simulink model "C_Sim"  (R2020b)
settings: Solver=ode4  StartTime=0.0  StopTime=t_f  FixedStep=dt  RelTol=1e-3
undefined symbols (not defined in the file or in its folder): A, B, K, Q, R, X0
settings Model: Creator=vahed  LastModifiedBy=vahed
settings DataIOCC: ReturnWorkspaceOutputs=off

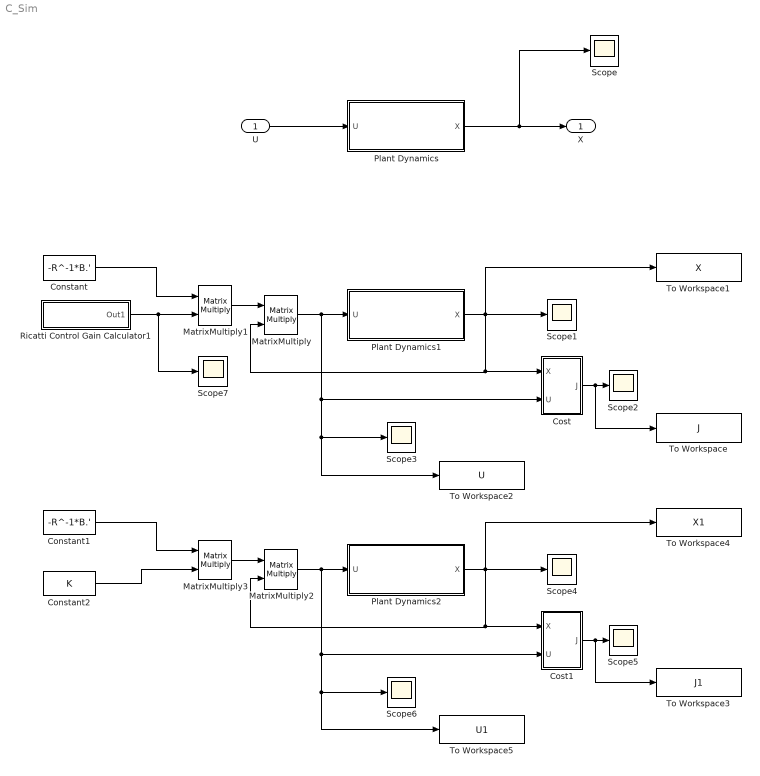
== system C_Sim ==
  U : Inport
  Constant : Constant  Value=-R^-1*B.'  VectorParams1D=off
  Constant1 : Constant  Value=-R^-1*B.'  VectorParams1D=off
  Constant2 : Constant  Value=K  VectorParams1D=off
  Cost : Subsystem
  Cost1 : Subsystem
  MatrixMultiply{,1..3} (4 alike) : Product  Multiplication=Matrix(*)
  Plant Dynamics : Subsystem
  Plant Dynamics1 : Subsystem
  Plant Dynamics2 : Subsystem
  Ricatti Control Gain Calculator1 : Subsystem
  Scope{,1..7} (8 alike) : Scope
  To Workspace : ToWorkspace  VariableName=J  SaveFormat=Structure With Time  SampleTime=-1
  To Workspace1 : ToWorkspace  VariableName=X  SaveFormat=Structure With Time  SampleTime=-1
  To Workspace2 : ToWorkspace  VariableName=U  SaveFormat=Structure With Time  SampleTime=-1
  To Workspace3 : ToWorkspace  VariableName=J1  SaveFormat=Structure With Time  SampleTime=-1
  To Workspace4 : ToWorkspace  VariableName=X1  SaveFormat=Structure With Time  SampleTime=-1
  To Workspace5 : ToWorkspace  VariableName=U1  SaveFormat=Structure With Time  SampleTime=-1
  X : Outport
  wires:
  U/1 -> Plant Dynamics/1(U)
  Plant Dynamics/1(X) -> Scope/1, X/1
  MatrixMultiply1/1 -> MatrixMultiply/1
  Ricatti Control Gain Calculator1/1(Out1) -> Scope7/1, MatrixMultiply1/2
  Constant/1 -> MatrixMultiply1/1
  Plant Dynamics1/1(X) -> MatrixMultiply/2, Cost/1(X), To Workspace1/1, Scope1/1
  MatrixMultiply/1 -> Scope3/1, To Workspace2/1, Cost/2(U), Plant Dynamics1/1(U)
  Cost/1(J) -> To Workspace/1, Scope2/1
  Cost1/1(J) -> Scope5/1, To Workspace3/1
  MatrixMultiply2/1 -> Plant Dynamics2/1(U), Cost1/2(U), To Workspace5/1, Scope6/1
  Plant Dynamics2/1(X) -> Scope4/1, To Workspace4/1, Cost1/1(X), MatrixMultiply2/2
  Constant1/1 -> MatrixMultiply3/1
  MatrixMultiply3/1 -> MatrixMultiply2/1
  Constant2/1 -> MatrixMultiply3/2

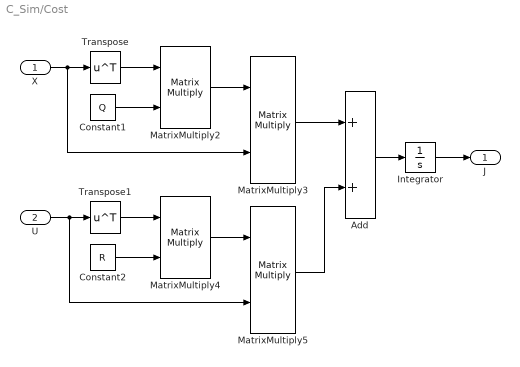
== system C_Sim/Cost ==
  X : Inport
  U : Inport  Port=2
  Add : Sum
  Constant1 : Constant  Value=Q  VectorParams1D=off
  Constant2 : Constant  Value=R  VectorParams1D=off
  Integrator : Integrator
  MatrixMultiply{2..5} (4 alike) : Product  Multiplication=Matrix(*)
  Transpose : Math  Operator=transpose  SaturateOnIntegerOverflow=on
  Transpose1 : Math  Operator=transpose  SaturateOnIntegerOverflow=on
  J : Outport
  wires:
  Constant1/1 -> MatrixMultiply2/2
  MatrixMultiply2/1 -> MatrixMultiply3/1
  MatrixMultiply3/1 -> Add/1
  U/1 -> MatrixMultiply5/2, Transpose1/1
  Transpose/1 -> MatrixMultiply2/1
  Add/1 -> Integrator/1
  MatrixMultiply4/1 -> MatrixMultiply5/1
  Transpose1/1 -> MatrixMultiply4/1
  Constant2/1 -> MatrixMultiply4/2
  Integrator/1 -> J/1
  MatrixMultiply5/1 -> Add/2
  X/1 -> MatrixMultiply3/2, Transpose/1

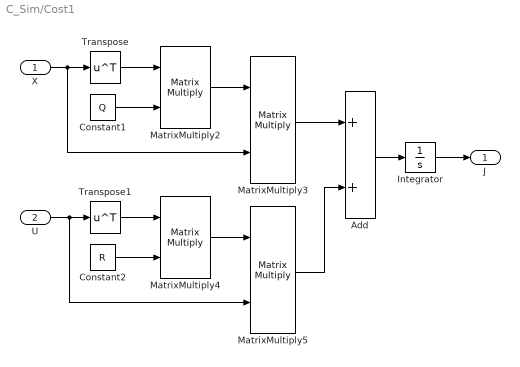
== system C_Sim/Cost1 ==
  X : Inport
  U : Inport  Port=2
  Add : Sum
  Constant1 : Constant  Value=Q  VectorParams1D=off
  Constant2 : Constant  Value=R  VectorParams1D=off
  Integrator : Integrator
  MatrixMultiply{2..5} (4 alike) : Product  Multiplication=Matrix(*)
  Transpose : Math  Operator=transpose  SaturateOnIntegerOverflow=on
  Transpose1 : Math  Operator=transpose  SaturateOnIntegerOverflow=on
  J : Outport
  wires:
  X/1 -> Transpose/1, MatrixMultiply3/2
  MatrixMultiply5/1 -> Add/2
  Integrator/1 -> J/1
  Constant2/1 -> MatrixMultiply4/2
  Transpose1/1 -> MatrixMultiply4/1
  MatrixMultiply4/1 -> MatrixMultiply5/1
  Add/1 -> Integrator/1
  Transpose/1 -> MatrixMultiply2/1
  U/1 -> Transpose1/1, MatrixMultiply5/2
  MatrixMultiply3/1 -> Add/1
  MatrixMultiply2/1 -> MatrixMultiply3/1
  Constant1/1 -> MatrixMultiply2/2

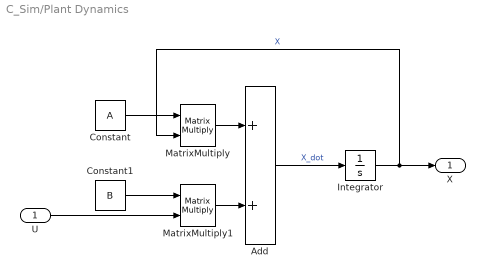
== system C_Sim/Plant Dynamics ==
  U : Inport
  Add : Sum
  Constant : Constant  Value=A  VectorParams1D=off
  Constant1 : Constant  Value=B  VectorParams1D=off
  Integrator : Integrator  InitialCondition=X0
  MatrixMultiply : Product  Multiplication=Matrix(*)
  MatrixMultiply1 : Product  Multiplication=Matrix(*)
  X : Outport
  wires:
  U/1 -> MatrixMultiply1/2
  Integrator/1 -> X/1, MatrixMultiply/2  "X"
  MatrixMultiply/1 -> Add/1
  Add/1 -> Integrator/1  "X_dot"
  Constant1/1 -> MatrixMultiply1/1
  MatrixMultiply1/1 -> Add/2
  Constant/1 -> MatrixMultiply/1

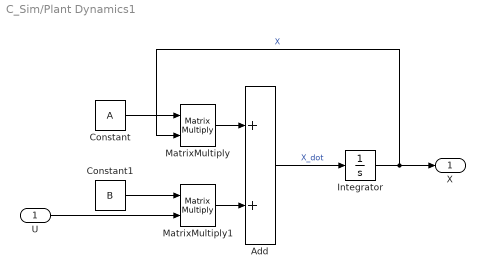
== system C_Sim/Plant Dynamics1 ==
  U : Inport
  Add : Sum
  Constant : Constant  Value=A
  Constant1 : Constant  Value=B
  Integrator : Integrator  InitialCondition=X0
  MatrixMultiply : Product  Multiplication=Matrix(*)
  MatrixMultiply1 : Product  Multiplication=Matrix(*)
  X : Outport
  wires:
  Constant/1 -> MatrixMultiply/1
  MatrixMultiply1/1 -> Add/2
  Constant1/1 -> MatrixMultiply1/1
  Add/1 -> Integrator/1  "X_dot"
  MatrixMultiply/1 -> Add/1
  Integrator/1 -> MatrixMultiply/2, X/1  "X"
  U/1 -> MatrixMultiply1/2

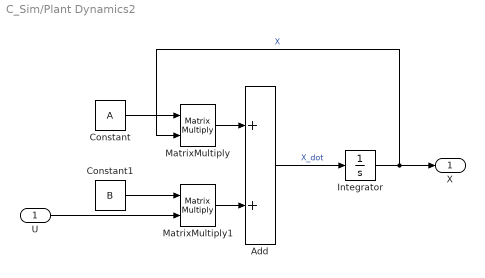
== system C_Sim/Plant Dynamics2 ==
  U : Inport
  Add : Sum
  Constant : Constant  Value=A
  Constant1 : Constant  Value=B
  Integrator : Integrator  InitialCondition=X0
  MatrixMultiply : Product  Multiplication=Matrix(*)
  MatrixMultiply1 : Product  Multiplication=Matrix(*)
  X : Outport
  wires:
  U/1 -> MatrixMultiply1/2
  Integrator/1 -> X/1, MatrixMultiply/2  "X"
  MatrixMultiply/1 -> Add/1
  Add/1 -> Integrator/1  "X_dot"
  Constant1/1 -> MatrixMultiply1/1
  MatrixMultiply1/1 -> Add/2
  Constant/1 -> MatrixMultiply/1

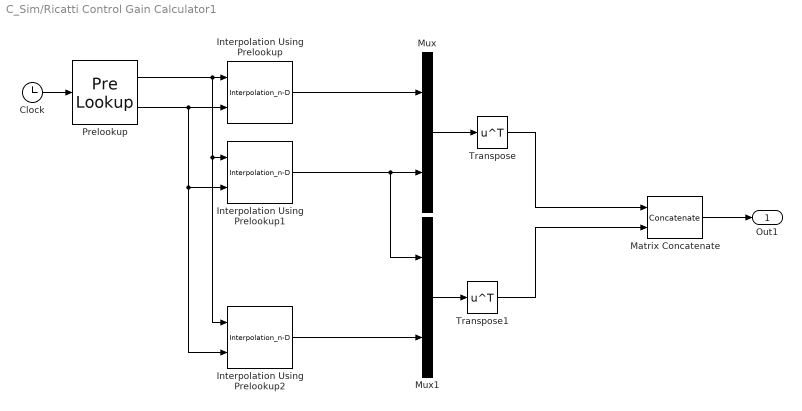
== system C_Sim/Ricatti Control Gain Calculator1 ==
  Clock : Clock
  Interpolation Using Prelookup : Interpolation_n-D  NumberOfTableDimensions=1  Table=Xx(end:-1:1,1)  ExtrapMethod=Clip  InternalRulePriority=Speed
      settings: InputPortMap=u0,u1
  Interpolation Using Prelookup1 : Interpolation_n-D  NumberOfTableDimensions=1  Table=Xx(end:-1:1,2)  ExtrapMethod=Clip  InternalRulePriority=Speed
      settings: InputPortMap=u0,u1
  Interpolation Using Prelookup2 : Interpolation_n-D  NumberOfTableDimensions=1  Table=Xx(end:-1:1,4)  ExtrapMethod=Clip  InternalRulePriority=Speed
      settings: InputPortMap=u0,u1
  Matrix Concatenate : Concatenate  Mode=Multidimensional array
  Mux : Mux  Inputs=2
  Mux1 : Mux  Inputs=2
  Prelookup : PreLookup  BreakpointsData=T
  Transpose : Math  Operator=transpose  SaturateOnIntegerOverflow=on
  Transpose1 : Math  Operator=transpose  SaturateOnIntegerOverflow=on
  Out1 : Outport
  wires:
  Prelookup/1 -> Interpolation Using Prelookup2/1, Interpolation Using Prelookup1/1, Interpolation Using Prelookup/1
  Clock/1 -> Prelookup/1
  Prelookup/2 -> Interpolation Using Prelookup2/2, Interpolation Using Prelookup1/2, Interpolation Using Prelookup/2
  Interpolation Using Prelookup/1 -> Mux/1
  Interpolation Using Prelookup1/1 -> Mux1/1, Mux/2
  Mux/1 -> Transpose/1
  Matrix Concatenate/1 -> Out1/1
  Interpolation Using Prelookup2/1 -> Mux1/2
  Mux1/1 -> Transpose1/1
  Transpose/1 -> Matrix Concatenate/1
  Transpose1/1 -> Matrix Concatenate/2
